simulink model "modules_intentions"  (R2017a)
settings: Solver=ode4  StartTime=0.0  StopTime=time_stop  FixedStep=time_step  RelTol=1e-3
undefined symbols (not defined in the file or in its folder): beta, Delta_guidance, Delta_matrix, eta_initial, initial_desired_psi_vector, initial_desired_u_vector, initial_next_waypoint_indexes, initial_obstacle_ship_states, initial_obstacle_ship_states_dot, initial_reference_psi_vector, initial_reference_u_vector, initial_SBMPC_desired_psi_vector, initial_SBMPC_desired_u_vector, initial_SBMPC_next_waypoint_indexes, initial_SBMPC_obstacle_ship_states, initial_SBMPC_obstacle_ship_states_dot, initial_SBMPC_reference_psi_vector, initial_SBMPC_reference_u_vector, initial_SBMPC_x_d_psi_matrix, initial_SBMPC_x_d_u_matrix, initial_state, initial_x_d_psi_matrix, initial_x_d_u_matrix, K_sway, K_yaw, Kp_feedback_linearization, kp_heading, Nmax, nu_initial, num_obs_ship_waypoints, num_prediction_time_steps, number_of_control_behaviors, number_of_obstacle_ships, number_of_SBMPC_obstacle_ships, obs_speed_between_waypoints, obstacle_waypoint_matrix, Omega_matrix, own_ship_reference_psi_init, own_ship_reference_speed, psi, Psi_init, radius_of_acceptance, SBMPC_obs_speed_between_waypoints, SBMPC_obstacle_waypoint_matrix, seconds_between_prediction, state_vector_init, T, T_k_surge, T_k_sway, T_k_yaw, T_s, T_waypoints, time_step, tsamp, U, U_init, V_init, waypoints_obstacle_ships, waypoints_own_ship, Xmax ... (+1)
(part 6 of 6)

== matlab function modules_intentions/Own-ship/SBMPC USING INTENTIONS /Normal obstacle ships trajectories prediction without intentions /Normal obstacle ships trajectories prediction without intentions ==
  settings: updateMethod=DISCRETE  sampleTime=time_step
  data: obstacle_ships_headings input; obstacle_ships_x_predicted output size=[num_prediction_time_steps, number_of_obstacle_ships]; obstacle_ships_y_predicted output size=[num_prediction_time_steps, number_of_obstacle_ships]; obstacle_ships_next_waypoint_index_vector input; obstacle_ships_initial_positions input; obstacle_ships_u input; obstacle_ships_v input; T_s parameter; t_0 input; number_of_obstacle_ships parameter; seconds_between_prediction parameter; num_prediction_time_steps parameter; obstacle_ships_u_predicted output size=[num_prediction_time_steps, number_of_obstacle_ships]; obstacle_ships_v_predicted output size=[num_prediction_time_steps, number_of_obstacle_ships]; obstacle_ships_psi_predicted output size=[num_prediction_time_steps, number_of_obstacle_ships]
function [obstacle_ships_x_predicted,obstacle_ships_y_predicted, obstacle_ships_u_predicted, obstacle_ships_v_predicted, obstacle_ships_psi_predicted] = normalObstacleShipsTrajectoryPrediction(obstacle_ships_headings, obstacle_ships_next_waypoint_index_vector, obstacle_ships_initial_positions, obstacle_ships_u, obstacle_ships_v, T_s, t_0, number_of_obstacle_ships, seconds_between_prediction, num_prediction_time_steps)
     deg2rad = pi/180;
     rad2deg = 180/pi;
     obstacle_ships_x_predicted = zeros( num_prediction_time_steps, number_of_obstacle_ships);   % obstacle_ships_x_predicted_init;  %%each row is a point in time, each column is an obstacle
     obstacle_ships_y_predicted = zeros( num_prediction_time_steps, number_of_obstacle_ships);   %obstacle_ships_y_predicted_init;  %%each row is a point in time, each column is an obstacle    
     obstacle_ships_u_predicted = zeros( num_prediction_time_steps, number_of_obstacle_ships);
     obstacle_ships_v_predicted = zeros( num_prediction_time_steps, number_of_obstacle_ships);
     obstacle_ships_psi_predicted = zeros( num_prediction_time_steps, number_of_obstacle_ships);
     if (mod(t_0, seconds_between_prediction) == 0)                 %Only do calculation every "seconds_between_prediction" second.
         for obstacle_ship_index = 1:number_of_obstacle_ships
             obstacle_ships_x_predicted(1, obstacle_ship_index) = obstacle_ships_initial_positions(obstacle_ship_index, 1);
             obstacle_ships_y_predicted(1, obstacle_ship_index) = obstacle_ships_initial_positions(obstacle_ship_index, 2);
             obstacle_ships_u_predicted(1, obstacle_ship_index) =obstacle_ships_u(obstacle_ship_index);
             obstacle_ships_v_predicted(1, obstacle_ship_index) = obstacle_ships_v(obstacle_ship_index);
             obstacle_ships_psi_predicted(1, obstacle_ship_index) = obstacle_ships_headings(obstacle_ship_index);
             for i = 2:num_prediction_time_steps
                obstacle_ship_speed = sqrt(obstacle_ships_u(obstacle_ship_index)^2 + obstacle_ships_v(obstacle_ship_index)^2);
                obstacle_ships_u_predicted(i,obstacle_ship_index) = obstacle_ships_u(obstacle_ship_index); %assume same speed for entire prediction horizon
                obstacle_ships_v_predicted(i,obstacle_ship_index) = obstacle_ships_v(obstacle_ship_index);
                obstacle_ships_psi_predicted(i, obstacle_ship_index) = obstacle_ships_headings(obstacle_ship_index);
                obstacle_ships_x_predicted(i,obstacle_ship_index) = obstacle_ships_x_predicted(i-1,obstacle_ship_index) + obstacle_ship_speed*cos(obstacle_ships_headings(obstacle_ship_index))*(T_s);   
                obstacle_ships_y_predicted(i,obstacle_ship_index) = obstacle_ships_y_predicted(i-1,obstacle_ship_index) + obstacle_ship_speed*sin(obstacle_ships_headings(obstacle_ship_index))*(T_s);
             end
             
         end % end for
     end % end if

end
